simulink model "problem6"  (R2020b)
settings: Solver=VariableStepAuto  StartTime=0.0  StopTime=10.0  RelTol=1e-3
settings Model: Creator=Shree  LastModifiedBy=Shree

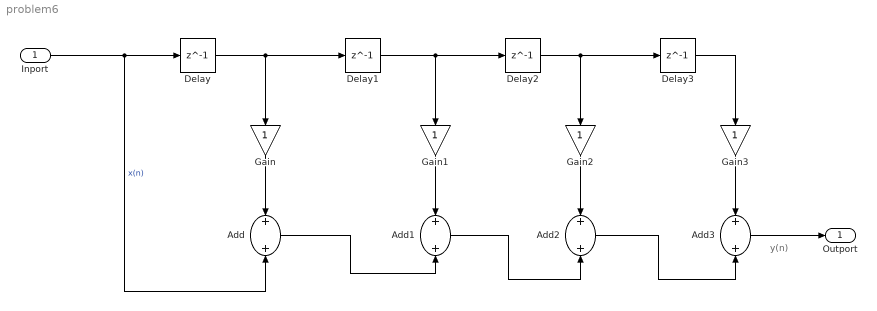
== system problem6 ==
  note: y(n)
  Inport : Inport
  Add{,1..3} (4 alike) : Sum
  Delay{,1..3} (4 alike) : Delay  DelayLength=1
  Gain{,1..3} (4 alike) : Gain
  Outport : Outport
  wires:
  Inport/1 -> Add/2, Delay/1  "x(n)"
  Delay/1 -> Gain/1, Delay1/1
  Delay1/1 -> Gain1/1, Delay2/1
  Delay2/1 -> Gain2/1, Delay3/1
  Gain1/1 -> Add1/1
  Gain/1 -> Add/1
  Gain2/1 -> Add2/1
  Gain3/1 -> Add3/1
  Add/1 -> Add1/2
  Add1/1 -> Add2/2
  Add2/1 -> Add3/2
  Delay3/1 -> Gain3/1
  Add3/1 -> Outport/1
